simulink model "CS2_Hzv"  (R2018b)
settings: Solver=VariableStepAuto  StartTime=0.0  StopTime=10.0  RelTol=1e-3
settings Model: Creator=bogda  LastModifiedBy=bogda

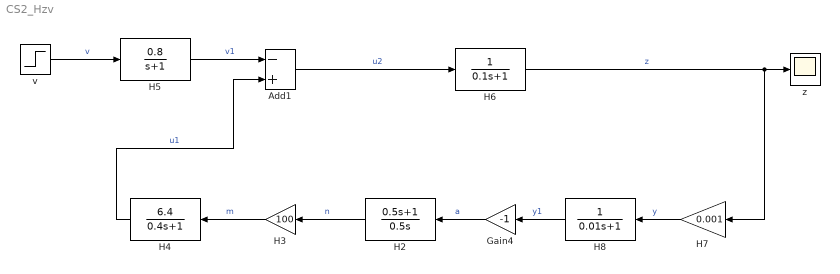
== system CS2_Hzv ==
  Add1 : Sum  Inputs=-+
  Gain4 : Gain  Gain=-1
  H2 : TransferFcn  Numerator=[0.5 1]  Denominator=[0.5 0]
  H3 : Gain  Gain=100
  H4 : TransferFcn  Numerator=[6.4]  Denominator=[0.4 1]
  H5 : TransferFcn  Numerator=[0.8]  Denominator=[1 1]
  H6 : TransferFcn  Denominator=[0.1 1]
  H7 : Gain  Gain=0.001
  H8 : TransferFcn  Denominator=[0.01 1]
  v : Step  Time=0  After=1250  SampleTime=0
  z : Scope
  wires:
  H7/1 -> H8/1  "y"
  H3/1 -> H4/1  "m"
  H5/1 -> Add1/1  "v1"
  H4/1 -> Add1/2  "u1"
  H8/1 -> Gain4/1  "y1"
  Gain4/1 -> H2/1  "a"
  v/1 -> H5/1  "v"
  H2/1 -> H3/1  "n"
  Add1/1 -> H6/1  "u2"
  H6/1 -> H7/1, z/1  "z"
